simulink model "MyKoshi"  (Simulink 7.9)
settings: Solver=ode45  StartTime=0.0  StopTime=50.0  RelTol=1e-3
libraries: simulink x2
settings Model: Creator=Mihail  LastModifiedBy=Mihail

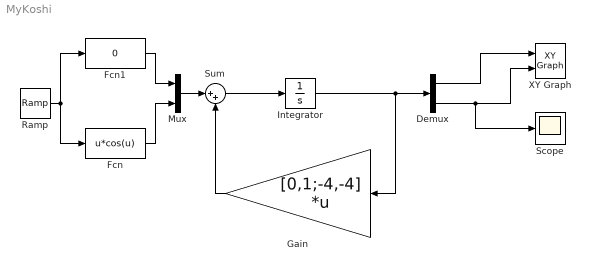
== system MyKoshi ==
  Demux : Demux  Outputs=2
  Fcn : Fcn  Expr=u*cos(u)
  Fcn1 : Fcn  Expr=0
  Gain : Gain  Gain=[0,1;-4,-4]  Multiplication=Matrix(K*u) (u vector)
  Integrator : Integrator
  Mux : Mux  Inputs=2
  Ramp : simulink/Sources/Ramp  slope=1  start=0  X0=0
  Scope : Scope
  Sum : Sum  Inputs=|++
  XY Graph : simulink/Sinks/XY Graph  xmin=-10  xmax=10  ymin=-10  ymax=10  st=0.01
  wires:
  Demux/2 -> Scope/1, XY Graph/2
  Demux/1 -> XY Graph/1
  Integrator/1 -> Demux/1, Gain/1
  Gain/1 -> Sum/2
  Sum/1 -> Integrator/1
  Mux/1 -> Sum/1
  Fcn1/1 -> Mux/1
  Fcn/1 -> Mux/2
  Ramp/1 -> Fcn/1, Fcn1/1
